simulink model "test1"  (R2017a)
settings: Solver=FixedStepAuto  StartTime=0.0  StopTime=3.0  FixedStep=0.001  RelTol=1e-3
settings Model: Creator=lzr96  LastModifiedBy=lzr96

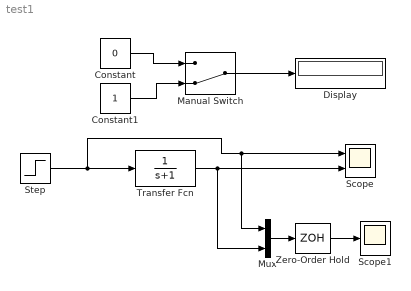
== system test1 ==
  Constant : Constant  Value=0
  Constant1 : Constant
  Display : Display
  Manual Switch : ManualSwitch  CurrentSetting=0
  Mux : Mux  Inputs=2
  Scope : Scope  NumInputPorts=2
  Scope1 : Scope
  Step : Step  SampleTime=0
  Transfer Fcn : TransferFcn  Denominator=[1 1]
  Zero-Order Hold : ZeroOrderHold  SampleTime=-1
  wires:
  Transfer Fcn/1 -> Mux/2, Scope/2
  Constant/1 -> Manual Switch/1
  Constant1/1 -> Manual Switch/2
  Manual Switch/1 -> Display/1
  Step/1 -> Mux/1, Scope/1, Transfer Fcn/1
  Mux/1 -> Zero-Order Hold/1
  Zero-Order Hold/1 -> Scope1/1
